simulink model "ME655_HW02"  (R2023a)
settings: Solver=ode45  StartTime=0.0  StopTime=t_f  RelTol=1e-3
values from neighbouring files (symbols this model uses):
  a3 = coefficients(1,1)    [ME655_HW02_Parameters.m]
  a4 = coefficients(2,1)    [ME655_HW02_Parameters.m]
  a5 = coefficients(3,1)    [ME655_HW02_Parameters.m]
  deltaP_error = [-.25;.05]    [ME655_HW02_Parameters.m]
  k_p = omega_n^2*eye(2)    [ME655_HW02_Parameters.m]
  k_v = 2*sqrt(k_p)*eye(2)    [ME655_HW02_Parameters.m]
  lc = 3    [ME655_HW02_Parameters.m]
  P_1 = [P_1x; P_1y]    [ME655_HW02_Parameters.m]
  P_2 = [P_2x; P_2y]    [ME655_HW02_Parameters.m]
  robot_geometry = [m1;m2;lc]    [ME655_HW02_Parameters.m]
settings Model: Creator=O135  LastModifiedBy=15512
settings SolverCC: AlgebraicLoopSolver=TrustRegion
settings DataIOCC: LimitDataPoints=on  SaveFormat=Array  ReturnWorkspaceOutputs=off
settings OptimizationCC: BlockReduction=off  BooleanDataType=off  LifeSpan=inf
settings DebuggingCC: SaveWithParameterizedLinksMsg=none  UnderspecifiedInitializationDetection=Classic  MergeDetectMultiDrivingBlocksExec=none  SignalResolutionControl=TryResolveAllWithWarning  UnconnectedInputMsg=warning  UnconnectedOutputMsg=warning  UnconnectedLineMsg=warning  SFUnexpectedBacktrackingDiag=warning  SFNoUnconditionalDefaultTransitionDiag=warning  SFExecutionAtInitializationDiag=none  ArithmeticOperatorsInVariantConditions=warning
settings HardwareCC: ProdBitPerPointer=32  ProdBitPerSizeT=32  ProdBitPerPtrDiffT=32  ProdLargestAtomicFloat=None  ProdIntDivRoundTo=Undefined  ProdEndianess=Unspecified  ProdWordSize=32  ProdHWDeviceType=32-bit Generic  TargetUnknown=on
settings ModelReferenceCC: EnableRefExpFcnMdlSchedulingChecks=on  PropagateSignalLabelsOutOfModel=off
settings SFSimCC: SimUseLocalCustomCode=off  CustomCodeUndefinedFunction=UseInterfaceOnly
settings RTWCC: RTWUseLocalCustomCode=off  DLArmComputeVersion=19.05
settings CodeAppCC: StateflowObjectComments=on
settings GRTTargetCC: TargetLangStandard=C89/C90 (ANSI)
settings ConfigComp: CovMetricSettings=dw  CovSaveCumulativeToWorkspaceVar=on  CovSaveSingleToWorkspaceVar=on  CovExternalEMLEnable=off  CovSFcnEnable=off

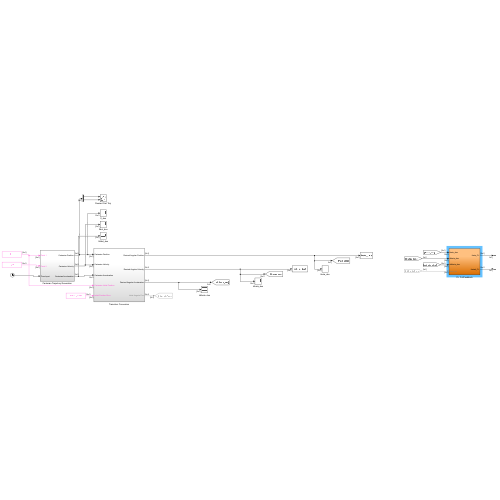
[thumbnail: Simulink's stored preview of the top-level diagram]
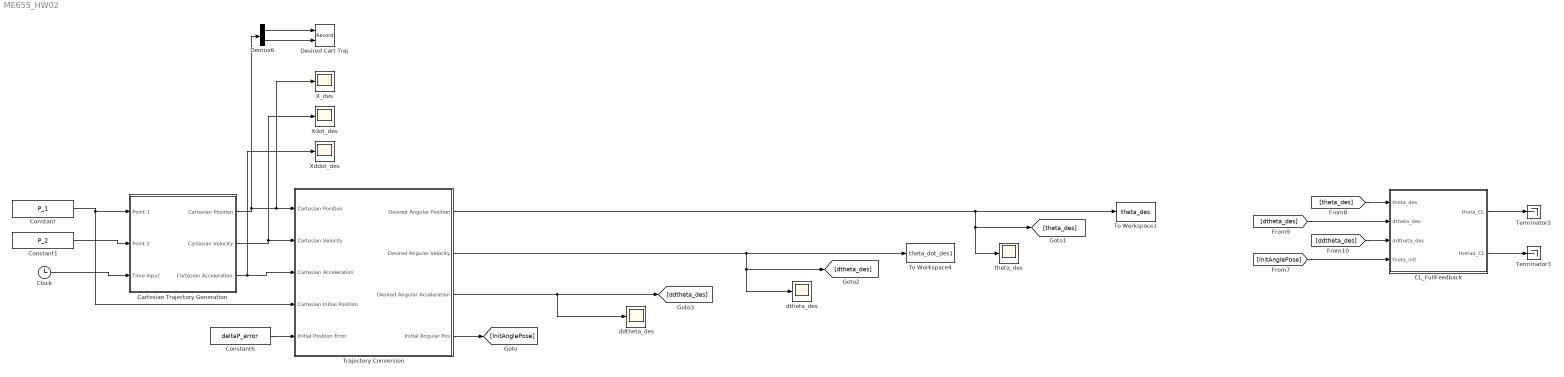
== system ME655_HW02 ==
  CL_FullFeedback : Subsystem
  Cartesian Trajectory Generation : Subsystem
  Clock : Clock
  Constant : Constant  Value=P_1  VectorParams1D=off
  Constant1 : Constant  Value=P_2  VectorParams1D=off
  Constant6 : Constant  Value=deltaP_error  VectorParams1D=off
  Demux6 : Demux  Outputs=2
  Desired Cart Traj : Record  FileSettingsInternal="{\"entries\":[{\"content\":{\"excelSettings\":{\"content\":{},\"type\":\"Streamout.ExcelSettings\"}},\"type\":\"Streamout.FileSettingStorage\",\"uuid\":\"575ce4a4-5469-47b1-a867-954e626e9ef8\"}],\"packageUris\":[\"http://schema.mathworks.com/mf0/streamout_blocks/R2020a\"],\"version\":\"1.0\"}"  Layout=[1 1]  SignalsInternal="{\"entries\":[{\"content\":{\"signals\":[{\"content\":{\"blockPath\":[\"ME655_HW02/Desired Cart Traj\"],\"dimensions\":[1,1],\"domain\":\"ME655_HW02/Desired Cart Traj\",\"lineColor\":\"#a2142f\",\"plots\":[1],\"port\":1,\"sid\":[\"\"],\"signalID\":313,\"signalName\":\"Demux6:1\"},\"type\":\"RecordBlkView.Signal\",\"uuid\":\"13b7ad26-6d5e-4f79-b7c3-48515e24de1a\"},{\"content\":{\"blockPath\":[\"ME655_HW02/Desired Cart Traj\"],\"dimensions\":[1,1],\"domain\":\"ME655_HW02/Desired Cart Traj\",\"lineColor\":\"#139fff\",\"plots\":[1],\"port\":2,\"sid\":[\"\"],\"signalID\":317,\"signalName\":\"Demux6:2\"},\"type\":\"RecordBlkView.Signal\",\"uuid\":\"80cb3473-6715-43ce-969d-17f6aacbd3f8\"}]},\"type\":\"RecordBlkView.InputSignals\",\"uuid\":\"c90513f2-26a6-43c8-9a7b-994466c783ed\"}],\"packageUris\":[\"http://schema.mathworks.com/mf0/streamout_blocks/R2020a\"],\"version\":\"1.0\"}"  VisualizationBindings="{\"xyplotplugin\":{\"info\":[{\"series\":[{\"bindingParametersList\":[{\"parameter\":\"X-Axis\",\"signalID\":313,\"signalName\":\"Demux6:1\"},{\"parameter\":\"Y-Axis\",\"signalID\":317,\"signalName\":\"Demux6:2\"}],\"seriesID\":13225}],\"subplotID\":1}]}}"  CompatibilityTag=XY  st=-1
  Terminator2 : Terminator
  Terminator3 : Terminator
  To Workspace1 : ToWorkspace  VariableName=theta_des  SaveFormat=Timeseries  SampleTime=-1
  To Workspace4 : ToWorkspace  VariableName=theta_dot_des1  SaveFormat=Timeseries  SampleTime=-1
  Trajectory Conversion : Subsystem
  X_des : Scope
  Xddot_des : Scope
  Xdot_des : Scope
  ddtheta_des : Scope
  dtheta_des : Scope
  theta_des : Scope
  wires:
  Constant/1 -> Trajectory Conversion/4(Cartesian Initial Position), Cartesian Trajectory Generation/1(Point 1)
  Constant1/1 -> Cartesian Trajectory Generation/2(Point 2)
  Clock/1 -> Cartesian Trajectory Generation/3(Time Input)
  Cartesian Trajectory Generation/1(Cartesian Position) -> Demux6/1, X_des/1, Trajectory Conversion/1(Cartesian Position)
  Cartesian Trajectory Generation/2(Cartesian Velocity) -> Xdot_des/1, Trajectory Conversion/2(Cartesian Velocity)
  Trajectory Conversion/2(Desired Angular Velocity) -> To Workspace4/1, [dtheta_des], dtheta_des/1
  Trajectory Conversion/3(Desired Angular Acceleration) -> [ddtheta_des], ddtheta_des/1
  Trajectory Conversion/4(Initial Angular Pos) -> [InitAnglePose]
  Trajectory Conversion/1(Desired Angular Position) -> [theta_des], theta_des/1, To Workspace1/1
  Demux6/1 -> Desired Cart Traj/1
  Demux6/2 -> Desired Cart Traj/2
  Constant6/1 -> Trajectory Conversion/5(Initial Position Error)
  CL_FullFeedback/1(theta_CL) -> Terminator2/1
  CL_FullFeedback/2(thetad_CL) -> Terminator3/1
  [dtheta_des] -> CL_FullFeedback/2(dtheta_des)
  [InitAnglePose] -> CL_FullFeedback/4(theta_init)
  [theta_des] -> CL_FullFeedback/1(theta_des)
  [ddtheta_des] -> CL_FullFeedback/3(ddtheta_des)
  Cartesian Trajectory Generation/3(Cartesian Acceleration) -> Xddot_des/1, Trajectory Conversion/3(Cartesian Acceleration)

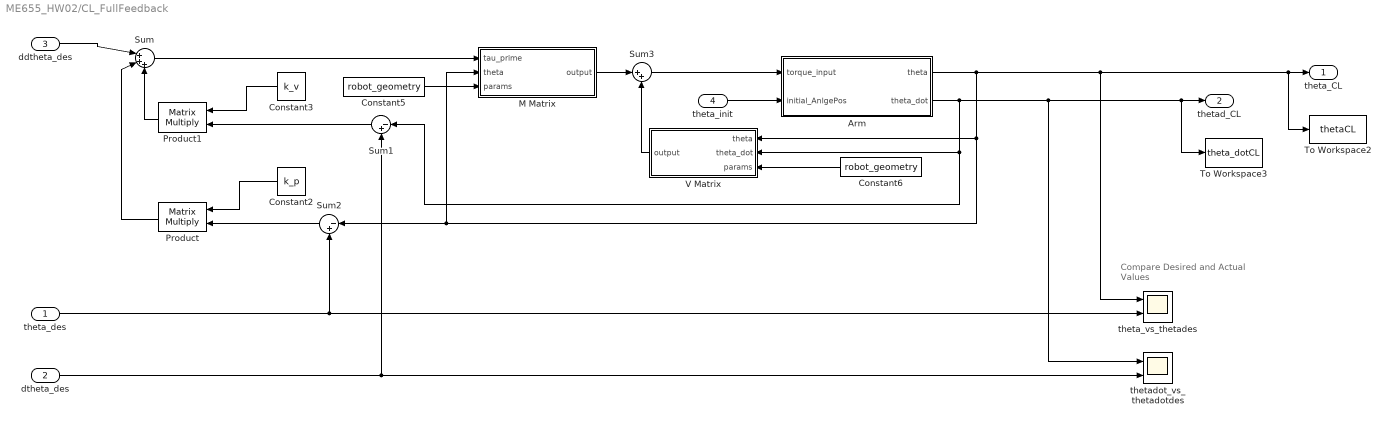
== system ME655_HW02/CL_FullFeedback ==
  note: Compare Desired
      | and Actual Values
  theta_des : Inport  PortDimensions=[2 1]
  dtheta_des : Inport  Port=2  PortDimensions=[2 1]
  ddtheta_des : Inport  Port=3  PortDimensions=[2 1]
  theta_init : Inport  Port=4  PortDimensions=[2 1]
  Arm : Subsystem
  Constant2 : Constant  Value=k_p
  Constant3 : Constant  Value=k_v
  Constant5 : Constant  Value=robot_geometry
  Constant6 : Constant  Value=robot_geometry
  M Matrix : MATLAB Function  TreatAsAtomicUnit=on
  Product : Product  Multiplication=Matrix(*)
  Product1 : Product  Multiplication=Matrix(*)
  Sum : Sum  Inputs=|+++
  Sum1 : Sum  Inputs=|-+
  Sum2 : Sum  Inputs=|-+
  Sum3 : Sum  Inputs=|++  InputSameDT=on
  To Workspace2 : ToWorkspace  VariableName=thetaCL  SaveFormat=Timeseries  SampleTime=-1
  To Workspace3 : ToWorkspace  VariableName=theta_dotCL  SaveFormat=Timeseries  SampleTime=-1
  V Matrix : MATLAB Function  TreatAsAtomicUnit=on
  theta_vs_thetades : Scope  NumInputPorts=2
  thetadot_vs_thetadotdes : Scope  NumInputPorts=2
  theta_CL : Outport  PortDimensions=[2 1]
  thetad_CL : Outport  Port=2  PortDimensions=[2 1]
  wires:
  Sum/1 -> M Matrix/1(tau_prime)
  M Matrix/1(output) -> Sum3/1
  Product/1 -> Sum/2
  Product1/1 -> Sum/3
  theta_init/1 -> Arm/2(initial_AnlgePos)
  Arm/2(theta_dot) -> To Workspace3/1, thetad_CL/1, thetadot_vs_thetadotdes/1, Sum1/1, V Matrix/2(theta_dot)
  V Matrix/1(output) -> Sum3/2
  dtheta_des/1 -> Sum1/2, thetadot_vs_thetadotdes/2
  Constant5/1 -> M Matrix/3(params)
  Sum3/1 -> Arm/1(torque_input)
  theta_des/1 -> Sum2/2, theta_vs_thetades/2
  Arm/1(theta) -> To Workspace2/1, theta_CL/1, theta_vs_thetades/1, M Matrix/2(theta), Sum2/1, V Matrix/1(theta)
  Constant2/1 -> Product/1
  Sum2/1 -> Product/2
  Sum1/1 -> Product1/2
  Constant3/1 -> Product1/1
  Constant6/1 -> V Matrix/3(params)
  ddtheta_des/1 -> Sum/1

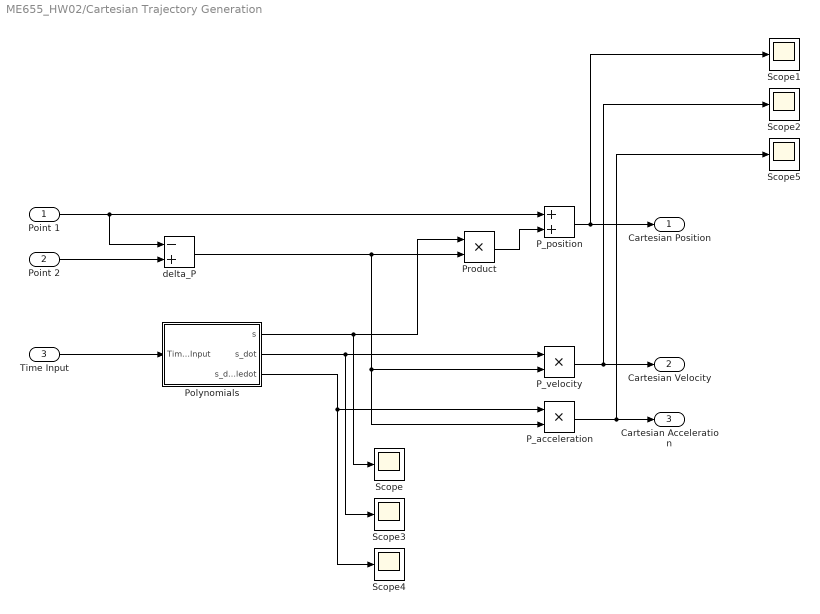
== system ME655_HW02/Cartesian Trajectory Generation ==
  Point 1 : Inport  PortDimensions=[2 1]
  Point 2 : Inport  Port=2  PortDimensions=[2 1]
  Time Input : Inport  Port=3
  P_acceleration : Product
  P_position : Sum
  P_velocity : Product
  Polynomials : Subsystem
  Product : Product
  Scope{,1..5} (6 alike) : Scope
  delta_P : Sum  Inputs=-+
  Cartesian Position : Outport
  Cartesian Velocity : Outport  Port=2
  Cartesian Acceleration : Outport  Port=3
  wires:
  Point 2/1 -> delta_P/2
  Polynomials/3(s_doubledot) -> Scope4/1, P_acceleration/1
  Point 1/1 -> P_position/1, delta_P/1
  Polynomials/2(s_dot) -> Scope3/1, P_velocity/1
  Polynomials/1(s) -> Scope/1, Product/1
  Time Input/1 -> Polynomials/1(Time Input)
  delta_P/1 -> P_acceleration/2, P_velocity/2, Product/2
  Product/1 -> P_position/2
  P_position/1 -> Scope1/1, Cartesian Position/1
  P_acceleration/1 -> Scope5/1, Cartesian Acceleration/1
  P_velocity/1 -> Scope2/1, Cartesian Velocity/1

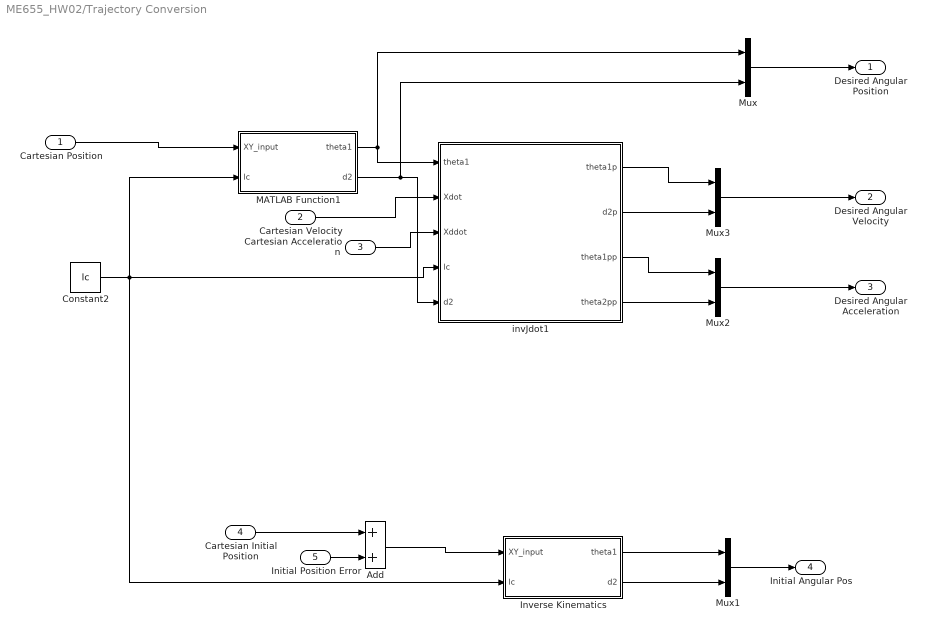
== system ME655_HW02/Trajectory Conversion ==
  Cartesian Position : Inport  PortDimensions=[2 1]
  Cartesian Velocity : Inport  Port=2  PortDimensions=[2 1]
  Cartesian Acceleration : Inport  Port=3  PortDimensions=[2 1]
  Cartesian Initial Position : Inport  Port=4  PortDimensions=[2 1]
  Initial Position Error : Inport  Port=5  PortDimensions=[2 1]
  Add : Sum
  Constant2 : Constant  Value=lc
  Inverse Kinematics : MATLAB Function  TreatAsAtomicUnit=on
  MATLAB Function1 : MATLAB Function  TreatAsAtomicUnit=on
  Mux{,1..3} (4 alike) : Mux  Inputs=2
  invJdot1 : MATLAB Function  TreatAsAtomicUnit=on
  Desired Angular Position : Outport  PortDimensions=[2 1]
  Desired Angular Velocity : Outport  Port=2  PortDimensions=[2 1]
  Desired Angular Acceleration : Outport  Port=3  PortDimensions=[2 1]
  Initial Angular Pos : Outport  Port=4  PortDimensions=[2 1]
  wires:
  MATLAB Function1/1(theta1) -> invJdot1/1(theta1), Mux/1
  MATLAB Function1/2(d2) -> invJdot1/5(d2), Mux/2
  Cartesian Position/1 -> MATLAB Function1/1(XY_input)
  Mux/1 -> Desired Angular Position/1
  Mux1/1 -> Initial Angular Pos/1
  Cartesian Velocity/1 -> invJdot1/2(Xdot)
  Cartesian Acceleration/1 -> invJdot1/3(Xddot)
  invJdot1/1(theta1p) -> Mux3/1
  invJdot1/2(d2p) -> Mux3/2
  invJdot1/3(theta1pp) -> Mux2/1
  invJdot1/4(theta2pp) -> Mux2/2
  Mux3/1 -> Desired Angular Velocity/1
  Mux2/1 -> Desired Angular Acceleration/1
  Constant2/1 -> MATLAB Function1/2(lc), Inverse Kinematics/2(lc), invJdot1/4(lc)
  Add/1 -> Inverse Kinematics/1(XY_input)
  Inverse Kinematics/2(d2) -> Mux1/2
  Inverse Kinematics/1(theta1) -> Mux1/1
  Cartesian Initial Position/1 -> Add/1
  Initial Position Error/1 -> Add/2

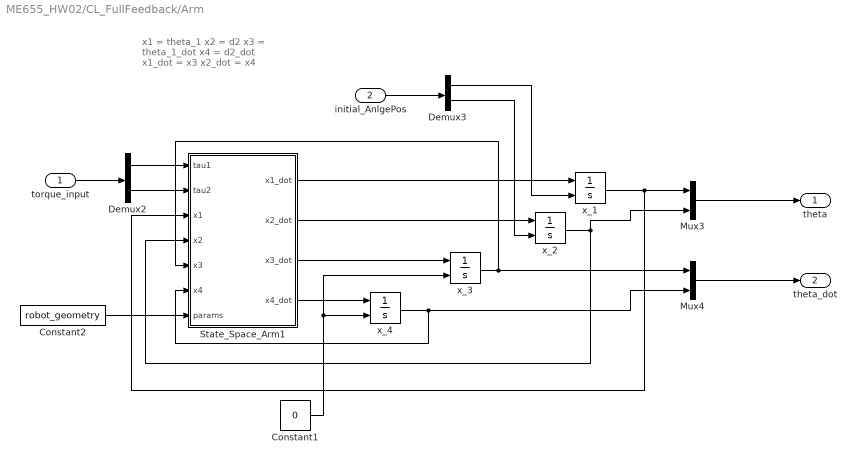
== system ME655_HW02/CL_FullFeedback/Arm ==
  note: x1 = theta_1
      | x2 = d2
      | x3 = theta_1_dot
      | x4 = d2_dot
      |
      | x1_dot = x3
      | x2_dot = x4
  torque_input : Inport  PortDimensions=[2 1]
  initial_AnlgePos : Inport  Port=2  PortDimensions=[2 1]
  Constant1 : Constant  Value=0
  Constant2 : Constant  Value=robot_geometry
  Demux2 : Demux  Outputs=2
  Demux3 : Demux  Outputs=2
  Mux3 : Mux  Inputs=2
  Mux4 : Mux  Inputs=2
  State_Space_Arm1 : MATLAB Function  TreatAsAtomicUnit=on
  x_{1..4} (4 alike) : Integrator  InitialConditionSource=external
  theta : Outport  PortDimensions=[2 1]
  theta_dot : Outport  Port=2  PortDimensions=[2 1]
  wires:
  State_Space_Arm1/1(x1_dot) -> x_1/1
  Constant1/1 -> x_3/2, x_4/2
  Demux2/1 -> State_Space_Arm1/1(tau1)
  x_1/1 -> Mux3/1, State_Space_Arm1/3(x1)
  State_Space_Arm1/3(x3_dot) -> x_3/1
  Demux2/2 -> State_Space_Arm1/2(tau2)
  x_2/1 -> Mux3/2, State_Space_Arm1/4(x2)
  Demux3/1 -> x_1/2
  State_Space_Arm1/4(x4_dot) -> x_4/1
  x_4/1 -> Mux4/2, State_Space_Arm1/6(x4)
  State_Space_Arm1/2(x2_dot) -> x_2/1
  Demux3/2 -> x_2/2
  x_3/1 -> State_Space_Arm1/5(x3), Mux4/1
  Mux4/1 -> theta_dot/1
  Mux3/1 -> theta/1
  initial_AnlgePos/1 -> Demux3/1
  torque_input/1 -> Demux2/1
  Constant2/1 -> State_Space_Arm1/7(params)

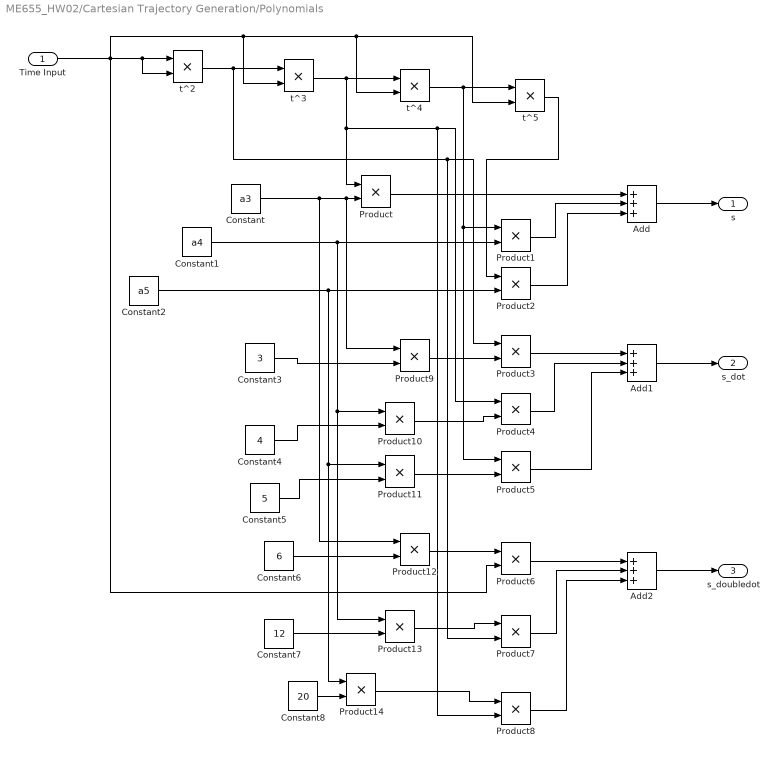
== system ME655_HW02/Cartesian Trajectory Generation/Polynomials ==
  Time Input : Inport
  Add : Sum  Inputs=+++
  Add1 : Sum  Inputs=+++
  Add2 : Sum  Inputs=+++
  Constant : Constant  Value=a3
  Constant1 : Constant  Value=a4
  Constant2 : Constant  Value=a5
  Constant3 : Constant  Value=3
  Constant4 : Constant  Value=4
  Constant5 : Constant  Value=5
  Constant6 : Constant  Value=6
  Constant7 : Constant  Value=12
  Constant8 : Constant  Value=20
  Product{,1..14} (15 alike) : Product
  t^{2..5} (4 alike) : Product
  s : Outport
  s_dot : Outport  Port=2
  s_doubledot : Outport  Port=3
  wires:
  Product14/1 -> Product8/1
  Product12/1 -> Product6/1
  t^4/1 -> Product5/1, Product1/1, t^5/1
  Product8/1 -> Add2/3
  Product6/1 -> Add2/1
  Add2/1 -> s_doubledot/1
  Add1/1 -> s_dot/1
  Product13/1 -> Product7/1
  Product7/1 -> Add2/2
  Product5/1 -> Add1/3
  Product10/1 -> Product4/2
  Product4/1 -> Add1/2
  Product1/1 -> Add/2
  Time Input/1 -> Product6/2, t^5/2, t^4/2, t^3/2, t^2/2, t^2/1
  Product11/1 -> Product5/2
  Product/1 -> Add/1
  Constant/1 -> Product12/1, Product9/1, Product/2
  Product2/1 -> Add/3
  Constant2/1 -> Product14/1, Product11/1, Product2/2
  t^2/1 -> Product7/2, Product3/1, t^3/1
  Product3/1 -> Add1/1
  Constant1/1 -> Product13/1, Product10/1, Product1/2
  t^3/1 -> Product8/2, Product4/1, Product/1, t^4/1
  t^5/1 -> Product2/1
  Add/1 -> s/1
  Constant3/1 -> Product9/2
  Product9/1 -> Product3/2
  Constant4/1 -> Product10/2
  Constant5/1 -> Product11/2
  Constant6/1 -> Product12/2
  Constant7/1 -> Product13/2
  Constant8/1 -> Product14/2

== matlab function ME655_HW02/CL_FullFeedback/Arm/State_Space_Arm1 ==
  data: x1_dot output; x2_dot output; tau1 input; tau2 input; x3_dot output; x1 input; x2 input; x3 input; x4 input; x4_dot output; params input
function [x1_dot,x2_dot,x3_dot,x4_dot] = fun(tau1, tau2, x1,x2,x3,x4,params)

m1=params(1);
m2=params(2);
l1=params(3);
% m1 = 2;
% m2 = 2;
% l1 = 3;
% l2 = 3;

x1_dot=x3;

x2_dot=x4;

x3_dot = 3*tau1/(4*(m2*x2^2 + m1*l1^2)) - 3*x2*x4*m2*x3/(2*(m2*x2^2 + m1*l1^2));

x4_dot = x2*x3^2 + tau2/m2;

% x3_dot = 3*tau1/(4*(m2*x2^2 + m1*l1^2)) - 3*x2*x4*m2*x3/(2*(m2*x2^2 + m1*l1^2));
% 
% x4_dot = x2*x3^2 + tau2/m2;
end

== matlab function ME655_HW02/CL_FullFeedback/M Matrix ==
  data: tau_prime input; theta input; output output; params input
function output = fcn(tau_prime, theta,params)

m1=params(1);
m2=params(2);
l1=params(3);

% m1 = 2;
% m2 = 2;
% l1 = 3;
% l2 = 3;

d2=theta(2);
M_matrix=[[m1*l1^2 + (1/3)*m1*l1^2 + (1/3)*m2*d2^2 + m2*d2^2, 0];
    [0, m2]];

% M_matrix=[[m1*l1^2 + (1/3)*m1*l1^2 + (1/3)*m2*d2^2 + m2*d2^2, 0];
%     [0, m2]];

output = M_matrix * tau_prime;

== matlab function ME655_HW02/CL_FullFeedback/V Matrix ==
  data: theta input; theta_dot input; output output; params input
function output  = fcn(theta, theta_dot,params)

m1=params(1);
m2=params(2);
l1=params(3);
% m1 = 2;
% m2 = 2;
% l1 = 3;
% l2 = 3;

d2=theta(2);
theta1p=theta_dot(1); d2p=theta_dot(2);

output =[2*m2*d2*theta1p*d2p;
    -m2*d2*theta1p^2];

% output =[2*m2*d2*theta1p*d2p;
%     -m2*d2*theta1p^2];

== matlab function ME655_HW02/Trajectory Conversion/Inverse Kinematics ==
  data: XY_input input; theta1 output; lc input; d2 output
function [theta1, d2] = fcn(XY_input, lc)

theta1 = atan2(XY_input(2),XY_input(1));
d2 = sqrt((XY_input(1))^2 + (XY_input(2))^2) - lc;

== matlab function ME655_HW02/Trajectory Conversion/MATLAB Function1 ==
  data: XY_input input; theta1 output; lc input; d2 output
function [theta1, d2] = fcn(XY_input, lc)

theta1 = atan2(XY_input(2),XY_input(1));
d2 = sqrt((XY_input(1))^2 + (XY_input(2))^2) - lc;

== matlab function ME655_HW02/Trajectory Conversion/invJdot1 ==
  data: theta1p output; d2p output; theta1 input; theta1pp output; Xdot input; Xddot input; theta2pp output; lc input; d2 input
function [theta1p,d2p,theta1pp,theta2pp]  = fcn(theta1,Xdot,Xddot,lc, d2)
%#codegen
thetap=invJ(theta1,d2,lc)*Xdot;
theta1p=thetap(1); d2p=thetap(2);
thetapp=invJ(theta1,d2,lc)*Xddot+invJdot(theta1,d2,theta1p,d2p,lc)*Xdot;
theta1pp=thetapp(1);theta2pp=thetapp(2);

end

function out  = invJ(theta1,d2,lc)
%#codegen
out=[[(-sin(theta1))/(d2+lc), (cos(theta1))/(d2+lc)];
    [cos(theta1), sin(theta1)]];
end

function out  = invJdot(theta1,d2,theta1p,d2p,lc)
%#codegen
out=[[d2p*((sin(theta1))/(d2+lc)^2) - theta1p*((cos(theta1))/(d2+lc)), -((cos(theta1))/(d2+lc)^2)*d2p];
[(sin(theta1))*theta1p, (cos(theta1))*theta1p]];
end
